simulink model "Boeing787_NewMission_ElectricalThermal"  (R2016a)
(part 7 of 17)

      | value = get_param(blk,'vel') ;
      | cellarr = get_param(blk,'MaskVisibilities') ;
      | ind = [1 4 9 12 15 18 21 24 27 30 33 38 43] ;
      | if strcmp(value,'on')
      |     cellarr(ind) = {'off'} ; cellarr(33:37) = {'on'} ;
      |     value1 = get_param(blk,'fromlen') ;
      |     value2 = get_param(blk,'fromtime') ;
      |     value3 = get_param(blk,'tolen') ;
      |     value4 = get_param(blk,'totime') ;
      |     if strcmp(get_param(blk,'vel'),'on')
      |         switch value1
      |             case 'Millimeters'
      |                 name1 = 'mm/' ;
      |                 fcn1  = 'u(1)/1000' ;
      |             case 'Meters'
      |                 name1 = 'm/' ;
      |                 fcn1  = 'u(1)' ;
      |             case 'Kilometers'
      |                 name1 = 'km/' ;
      |                 fcn1  = 'u(1)*1000' ;
      |             case 'Inches'
      |                 name1 = 'in/' ;
      |                 fcn1  = 'u(1)/39.37008' ;
      |             case 'Feet'
      |                 name1 = 'ft/' ;
      |                 fcn1  = 'u(1)/3.28084';
      |             case 'Yards'
      |                 name1 = 'yd/' ;
      |                 fcn1  = 'u(1)*3/3.28084' ;
      |             case 'Miles'
      |                 name1 = 'mi/' ;
      |                 fcn1  = 'u(1)*1609.344' ;
      |             case 'Nautical Miles'
      |                 name1 = 'nmi/' ;
      |                 fcn1  = 'u(1)*1852' ;
      |         end
      |         switch value2
      |             case 'Millisecond'
      |                 name2 = 'ms' ;
      |                 fcn2  = '*1000'  ;
      |             case 'Second'
      |                 name2 = 's' ;
      |                 fcn2  = '' ;
      |             case 'Minute'
      |                 name2 = 'min' ;
      |                 fcn2  = '/60' ;
      |             case 'Hour'
      |                 name2 = 'hr' ;
      |                 fcn2  = '/3600' ;
      |         end
      |         switch value3
      |             case 'Millimeters'
      |                 name3 = 'mm/' ;
      |                 fcn3  = '*1000' ;
      |             case 'Meters'
      |                 name3 = 'm/' ;
      |                 fcn3  = '' ;
      |             case 'Kilometers'
      |                 name3 = 'km/' ;
      |                 fcn3  = '/1000' ;
      |             case 'Inches'
      |                 name3 = 'in/' ;
      |                 fcn3  = '*39.37008' ;
      |             case 'Feet'
      |                 name3 = 'ft/' ;
      |                 fcn3  = '*3.28084';
      |             case 'Yards'
      |                 name3 = 'yd/' ;
      |                 fcn3  = '/3*3.28084' ;
      |             case 'Miles'
      |                 name3 = 'mi/' ;
      |                 fcn3  = '/1609.344' ;
      |             case 'Nautical Miles'
      |                 name3 = 'nmi/' ;
      |                 fcn3  = '/1852' ;
      |         end
      |         switch value4
      |             case 'Millisecond'
      |                 name4 = 'ms' ;
      |                 fcn4  = '/1000'  ;
      |             case 'Second'
      |                 name4 = 's' ;
      |                 fcn4  = '' ;
      |             case 'Minute'
      |                 name4 = 'min' ;
      |                 fcn4  = '*60' ;
      |             case 'Hour'
      |                 name4 = 'hr' ;
      |                 fcn4  = '*3600' ;
      |         end
      |         expr = [fcn1 fcn2 fcn3 fcn4] ;
      |         %set_param(blk,'func',func) ;
      |         set_param([blk '/conv_fcn'],'expr',expr) ;
      |         str1 = ['% this block of text is updated via dialog callbacks'];
      |         str2 = [char(39) 'horizontalAlignment' char(39) ',' char(39) 'center' char(39) ',' char(39) 'texmode' char(39) ',' char(39) 'on' char(39)] ;
      |         name = [char(39) name1 name2 ' to ' name3 name4 char(39)] ;
      |         str = sprintf('%s\ntext(.5,.5,%s,%s)',str1,name,str2) ;
      |         set_param(blk,'MaskDisplay',str) ;
      |     end
      |     clear value1 value2 value3 value4 expr name1 name2 name3 name4 name fcn1 fcn2 fcn3 fcn4 str1 str2 str
      | 
      | else
      |     cellarr(34:37) = {'off'} ; val = get_param(blk,'MaskValues') ;
      |     for i=1:length(ind)
      |         a = findstr(val{ind(i)},'on') ;
      |         b(i) = isempty(a) ;
      |     end
      |     if isempty(find(b==0)) ;
      |         cellarr(ind) = {'on'} ;
      |     end
      | end
      | set_param(blk,'MaskVisibilities',cellarr) ;
      | clear blk value cellarr ind a b val i
      mask TypeOptions fromlen: Millimeters | Meters | Kilometers | Inches | Feet | Yards | Miles | Nautical Miles
      mask Callback fromlen:
      | blk = gcb ;
      | value1 = get_param(blk,'fromlen') ;
      | value2 = get_param(blk,'fromtime') ;
      | value3 = get_param(blk,'tolen') ;
      | value4 = get_param(blk,'totime') ;
      | if strcmp(get_param(blk,'vel'),'on')
      |     switch value1
      |         case 'Millimeters'
      |             name1 = 'mm/' ;
      |             fcn1  = 'u(1)/1000' ;
      |         case 'Meters'
      |             name1 = 'm/' ;
      |             fcn1  = 'u(1)' ;
      |         case 'Kilometers'
      |             name1 = 'km/' ;
      |             fcn1  = 'u(1)*1000' ;
      |         case 'Inches'
      |             name1 = 'in/' ;
      |             fcn1  = 'u(1)/39.37008' ;
      |         case 'Feet'
      |             name1 = 'ft/' ;
      |             fcn1  = 'u(1)/3.28084';
      |         case 'Yards'
      |             name1 = 'yd/' ;
      |             fcn1  = 'u(1)*3/3.28084' ;
      |         case 'Miles'
      |             name1 = 'mi/' ;
      |             fcn1  = 'u(1)*1609.344' ;
      |         case 'Nautical Miles'
      |             name1 = 'nmi/' ;
      |             fcn1  = 'u(1)*1852' ;
      |     end
      |     switch value2
      |         case 'Millisecond'
      |             name2 = 'ms' ;
      |             fcn2  = '*1000'  ;
      |         case 'Second'
      |             name2 = 's' ;
      |             fcn2  = '' ;
      |         case 'Minute'
      |             name2 = 'min' ;
      |             fcn2  = '/60' ;
      |         case 'Hour'
      |             name2 = 'hr' ;
      |             fcn2  = '/3600' ;
      |     end
      |     switch value3
      |         case 'Millimeters'
      |             name3 = 'mm/' ;
      |             fcn3  = '*1000' ;
      |         case 'Meters'
      |             name3 = 'm/' ;
      |             fcn3  = '' ;
      |         case 'Kilometers'
      |             name3 = 'km/' ;
      |             fcn3  = '/1000' ;
      |         case 'Inches'
      |             name3 = 'in/' ;
      |             fcn3  = '*39.37008' ;
      |         case 'Feet'
      |             name3 = 'ft/' ;
      |             fcn3  = '*3.28084';
      |         case 'Yards'
      |             name3 = 'yd/' ;
      |             fcn3  = '/3*3.28084' ;
      |         case 'Miles'
      |             name3 = 'mi/' ;
      |             fcn3  = '/1609.344' ;
      |         case 'Nautical Miles'
      |             name3 = 'nmi/' ;
      |             fcn3  = '/1852' ;
      |     end
      |     switch value4
      |         case 'Millisecond'
      |             name4 = 'ms' ;
      |             fcn4  = '/1000'  ;
      |         case 'Second'
      |             name4 = 's' ;
      |             fcn4  = '' ;
      |         case 'Minute'
      |             name4 = 'min' ;
      |             fcn4  = '*60' ;
      |         case 'Hour'
      |             name4 = 'hr' ;
      |             fcn4  = '*3600' ;
      |     end
      |     expr = [fcn1 fcn2 fcn3 fcn4] ;
      |     %set_param(blk,'func',func) ;
      |     set_param([blk '/conv_fcn'],'expr',expr) ;
      |     str1 = ['% this block of text is updated via dialog callbacks'];
      |     str2 = [char(39) 'horizontalAlignment' char(39) ',' char(39) 'center' char(39) ',' char(39) 'texmode' char(39) ',' char(39) 'on' char(39)] ;
      |     name = [char(39) name1 name2 ' to ' name3 name4 char(39)] ;
      |     str = sprintf('%s\ntext(.5,.5,%s,%s)',str1,name,str2) ;
      |     set_param(blk,'MaskDisplay',str) ;
      | end
      | clear blk value1 value2 value3 value4 expr name1 name2 name3 name4 name fcn1 fcn2 fcn3 fcn4 str1 str2 str
      mask TypeOptions fromtime: Millisecond | Second | Minute | Hour
      mask Callback fromtime:
      | blk = gcb ;
      | value1 = get_param(blk,'fromlen') ;
      | value2 = get_param(blk,'fromtime') ;
      | value3 = get_param(blk,'tolen') ;
      | value4 = get_param(blk,'totime') ;
      | if strcmp(get_param(blk,'vel'),'on')
      |     switch value1
      |         case 'Millimeters'
      |             name1 = 'mm/' ;
      |             fcn1  = 'u(1)/1000' ;
      |         case 'Meters'
      |             name1 = 'm/' ;
      |             fcn1  = 'u(1)' ;
      |         case 'Kilometers'
      |             name1 = 'km/' ;
      |             fcn1  = 'u(1)*1000' ;
      |         case 'Inches'
      |             name1 = 'in/' ;
      |             fcn1  = 'u(1)/39.37008' ;
      |         case 'Feet'
      |             name1 = 'ft/' ;
      |             fcn1  = 'u(1)/3.28084';
      |         case 'Yards'
      |             name1 = 'yd/' ;
      |             fcn1  = 'u(1)*3/3.28084' ;
      |         case 'Miles'
      |             name1 = 'mi/' ;
      |             fcn1  = 'u(1)*1609.344' ;
      |         case 'Nautical Miles'
      |             name1 = 'nmi/' ;
      |             fcn1  = 'u(1)*1852' ;
      |     end
      |     switch value2
      |         case 'Millisecond'
      |             name2 = 'ms' ;
      |             fcn2  = '*1000'  ;
      |         case 'Second'
      |             name2 = 's' ;
      |             fcn2  = '' ;
      |         case 'Minute'
      |             name2 = 'min' ;
      |             fcn2  = '/60' ;
      |         case 'Hour'
      |             name2 = 'hr' ;
      |             fcn2  = '/3600' ;
      |     end
      |     switch value3
      |         case 'Millimeters'
      |             name3 = 'mm/' ;
      |             fcn3  = '*1000' ;
      |         case 'Meters'
      |             name3 = 'm/' ;
      |             fcn3  = '' ;
      |         case 'Kilometers'
      |             name3 = 'km/' ;
      |             fcn3  = '/1000' ;
      |         case 'Inches'
      |             name3 = 'in/' ;
      |             fcn3  = '*39.37008' ;
      |         case 'Feet'
      |             name3 = 'ft/' ;
      |             fcn3  = '*3.28084';
      |         case 'Yards'
      |             name3 = 'yd/' ;
      |             fcn3  = '/3*3.28084' ;
      |         case 'Miles'
      |             name3 = 'mi/' ;
      |             fcn3  = '/1609.344' ;
      |         case 'Nautical Miles'
      |             name3 = 'nmi/' ;
      |             fcn3  = '/1852' ;
      |     end
      |     switch value4
      |         case 'Millisecond'
      |             name4 = 'ms' ;
      |             fcn4  = '/1000'  ;
      |         case 'Second'
      |             name4 = 's' ;
      |             fcn4  = '' ;
      |         case 'Minute'
      |             name4 = 'min' ;
      |             fcn4  = '*60' ;
      |         case 'Hour'
      |             name4 = 'hr' ;
      |             fcn4  = '*3600' ;
      |     end
      |     expr = [fcn1 fcn2 fcn3 fcn4] ;
      |     %set_param(blk,'func',func) ;
      |     set_param([blk '/conv_fcn'],'expr',expr) ;
      |     str1 = ['% this block of text is updated via dialog callbacks'];
      |     str2 = [char(39) 'horizontalAlignment' char(39) ',' char(39) 'center' char(39) ',' char(39) 'texmode' char(39) ',' char(39) 'on' char(39)] ;
      |     name = [char(39) name1 name2 ' to ' name3 name4 char(39)] ;
      |     str = sprintf('%s\ntext(.5,.5,%s,%s)',str1,name,str2) ;
      |     set_param(blk,'MaskDisplay',str) ;
      | end
      | clear blk value1 value2 value3 value4 expr name1 name2 name3 name4 name fcn1 fcn2 fcn3 fcn4 str1 str2 str
      mask TypeOptions tolen: Millimeters | Meters | Kilometers | Inches | Feet | Yards | Miles | Nautical Miles
      mask Callback tolen:
      | blk = gcb ;
      | value1 = get_param(blk,'fromlen') ;
      | value2 = get_param(blk,'fromtime') ;
      | value3 = get_param(blk,'tolen') ;
      | value4 = get_param(blk,'totime') ;
      | if strcmp(get_param(blk,'vel'),'on')
      |     switch value1
      |         case 'Millimeters'
      |             name1 = 'mm/' ;
      |             fcn1  = 'u(1)/1000' ;
      |         case 'Meters'
      |             name1 = 'm/' ;
      |             fcn1  = 'u(1)' ;
      |         case 'Kilometers'
      |             name1 = 'km/' ;
      |             fcn1  = 'u(1)*1000' ;
      |         case 'Inches'
      |             name1 = 'in/' ;
      |             fcn1  = 'u(1)/39.37008' ;
      |         case 'Feet'
      |             name1 = 'ft/' ;
      |             fcn1  = 'u(1)/3.28084';
      |         case 'Yards'
      |             name1 = 'yd/' ;
      |             fcn1  = 'u(1)*3/3.28084' ;
      |         case 'Miles'
      |             name1 = 'mi/' ;
      |             fcn1  = 'u(1)*1609.344' ;
      |         case 'Nautical Miles'
      |             name1 = 'nmi/' ;
      |             fcn1  = 'u(1)*1852' ;
      |     end
      |     switch value2
      |         case 'Millisecond'
      |             name2 = 'ms' ;
      |             fcn2  = '*1000'  ;
      |         case 'Second'
      |             name2 = 's' ;
      |             fcn2  = '' ;
      |         case 'Minute'
      |             name2 = 'min' ;
      |             fcn2  = '/60' ;
      |         case 'Hour'
      |             name2 = 'hr' ;
      |             fcn2  = '/3600' ;
      |     end
      |     switch value3
      |         case 'Millimeters'
      |             name3 = 'mm/' ;
      |             fcn3  = '*1000' ;
      |         case 'Meters'
      |             name3 = 'm/' ;
      |             fcn3  = '' ;
      |         case 'Kilometers'
      |             name3 = 'km/' ;
      |             fcn3  = '/1000' ;
      |         case 'Inches'
      |             name3 = 'in/' ;
      |             fcn3  = '*39.37008' ;
      |         case 'Feet'
      |             name3 = 'ft/' ;
      |             fcn3  = '*3.28084';
      |         case 'Yards'
      |             name3 = 'yd/' ;
      |             fcn3  = '/3*3.28084' ;
      |         case 'Miles'
      |             name3 = 'mi/' ;
      |             fcn3  = '/1609.344' ;
      |         case 'Nautical Miles'
      |             name3 = 'nmi/' ;
      |             fcn3  = '/1852' ;
      |     end
      |     switch value4
      |         case 'Millisecond'
      |             name4 = 'ms' ;
      |             fcn4  = '/1000'  ;
      |         case 'Second'
      |             name4 = 's' ;
      |             fcn4  = '' ;
      |         case 'Minute'
      |             name4 = 'min' ;
      |             fcn4  = '*60' ;
      |         case 'Hour'
      |             name4 = 'hr' ;
      |             fcn4  = '*3600' ;
      |     end
      |     expr = [fcn1 fcn2 fcn3 fcn4] ;
      |     %set_param(blk,'func',func) ;
      |     set_param([blk '/conv_fcn'],'expr',expr) ;
      |     str1 = ['% this block of text is updated via dialog callbacks'];
      |     str2 = [char(39) 'horizontalAlignment' char(39) ',' char(39) 'center' char(39) ',' char(39) 'texmode' char(39) ',' char(39) 'on' char(39)] ;
      |     name = [char(39) name1 name2 ' to ' name3 name4 char(39)] ;
      |     str = sprintf('%s\ntext(.5,.5,%s,%s)',str1,name,str2) ;
      |     set_param(blk,'MaskDisplay',str) ;
      | end
      | clear blk value1 value2 value3 value4 expr name1 name2 name3 name4 name fcn1 fcn2 fcn3 fcn4 str1 str2 str
      mask TypeOptions totime: Millisecond | Second | Minute | Hour
      mask Callback totime:
      | blk = gcb ;
      | value1 = get_param(blk,'fromlen') ;
      | value2 = get_param(blk,'fromtime') ;
      | value3 = get_param(blk,'tolen') ;
      | value4 = get_param(blk,'totime') ;
      | if strcmp(get_param(blk,'vel'),'on')
      |     switch value1
      |         case 'Millimeters'
      |             name1 = 'mm/' ;
      |             fcn1  = 'u(1)/1000' ;
      |         case 'Meters'
      |             name1 = 'm/' ;
      |             fcn1  = 'u(1)' ;
      |         case 'Kilometers'
      |             name1 = 'km/' ;
      |             fcn1  = 'u(1)*1000' ;
      |         case 'Inches'
      |             name1 = 'in/' ;
      |             fcn1  = 'u(1)/39.37008' ;
      |         case 'Feet'
      |             name1 = 'ft/' ;
      |             fcn1  = 'u(1)/3.28084';
      |         case 'Yards'
      |             name1 = 'yd/' ;
      |             fcn1  = 'u(1)*3/3.28084' ;
      |         case 'Miles'
      |             name1 = 'mi/' ;
      |             fcn1  = 'u(1)*1609.344' ;
      |         case 'Nautical Miles'
      |             name1 = 'nmi/' ;
      |             fcn1  = 'u(1)*1852' ;
      |     end
      |     switch value2
      |         case 'Millisecond'
      |             name2 = 'ms' ;
      |             fcn2  = '*1000'  ;
      |         case 'Second'
      |             name2 = 's' ;
      |             fcn2  = '' ;
      |         case 'Minute'
      |             name2 = 'min' ;
      |             fcn2  = '/60' ;
      |         case 'Hour'
      |             name2 = 'hr' ;
      |             fcn2  = '/3600' ;
      |     end
      |     switch value3
      |         case 'Millimeters'
      |             name3 = 'mm/' ;
      |             fcn3  = '*1000' ;
      |         case 'Meters'
      |             name3 = 'm/' ;
      |             fcn3  = '' ;
      |         case 'Kilometers'
      |             name3 = 'km/' ;
      |             fcn3  = '/1000' ;
      |         case 'Inches'
      |             name3 = 'in/' ;
      |             fcn3  = '*39.37008' ;
      |         case 'Feet'
      |             name3 = 'ft/' ;
      |             fcn3  = '*3.28084';
      |         case 'Yards'
      |             name3 = 'yd/' ;
      |             fcn3  = '/3*3.28084' ;
      |         case 'Miles'
      |             name3 = 'mi/' ;
      |             fcn3  = '/1609.344' ;
      |         case 'Nautical Miles'
      |             name3 = 'nmi/' ;
      |             fcn3  = '/1852' ;
      |     end
      |     switch value4
      |         case 'Millisecond'
      |             name4 = 'ms' ;
      |             fcn4  = '/1000'  ;
      |         case 'Second'
      |             name4 = 's' ;
      |             fcn4  = '' ;
      |         case 'Minute'
      |             name4 = 'min' ;
      |             fcn4  = '*60' ;
      |         case 'Hour'
      |             name4 = 'hr' ;
      |             fcn4  = '*3600' ;
      |     end
      |     expr = [fcn1 fcn2 fcn3 fcn4] ;
      |     %set_param(blk,'func',func) ;
      |     set_param([blk '/conv_fcn'],'expr',expr) ;
      |     str1 = ['% this block of text is updated via dialog callbacks'];
      |     str2 = [char(39) 'horizontalAlignment' char(39) ',' char(39) 'center' char(39) ',' char(39) 'texmode' char(39) ',' char(39) 'on' char(39)] ;
      |     name = [char(39) name1 name2 ' to ' name3 name4 char(39)] ;
      |     str = sprintf('%s\ntext(.5,.5,%s,%s)',str1,name,str2) ;
      |     set_param(blk,'MaskDisplay',str) ;
      | end
      | clear blk value1 value2 value3 value4 expr name1 name2 name3 name4 name fcn1 fcn2 fcn3 fcn4 str1 str2 str
      mask Callback flow_rate:
      | blk = gcb ;
      | value = get_param(blk,'flow_rate') ;
      | cellarr = get_param(blk,'MaskVisibilities') ;
      | ind = [1 4 9 12 15 18 21 24 27 30 33 38 43] ;
      | if strcmp(value,'on')
      |     cellarr(ind) = {'off'} ; cellarr(38:42) = {'on'} ;
      |     value1 = get_param(blk,'fromflowvol') ;
      |     value2 = get_param(blk,'fromflvoltime') ;
      |     value3 = get_param(blk,'toflowvol') ;
      |     value4 = get_param(blk,'toflvoltime') ;
      |     if strcmp(get_param(blk,'flow_rate'),'on')
      |         switch value1
      |             case 'Milliliters'
      |                 name1 = 'mL/' ;
      |                 fcn1  = 'u(1)*(1e-6)' ;
      |             case 'Liters'
      |                 name1 = 'L/' ;
      |                 fcn1  = 'u(1)*.001' ;
      |             case 'Cubic Centimeters'
      |                 name1 = 'cm^3/' ;
      |                 fcn1  = 'u(1)*(1e-6)' ;
      |             case 'Cubic Meters'
      |                 name1 = 'm^3/' ;
      |                 fcn1  = 'u(1)' ;
      |             case 'Ounces'
      |                 name1 = 'oz/' ;
      |                 fcn1  = 'u(1)*(2.957353e-5)';
      |             case 'Gallons'
      |                 name1 = 'gal/' ;
      |                 fcn1  = 'u(1)*.00378541' ;
      |             case 'Cubic Inches'
      |                 name1 = 'in^3/' ;
      |                 fcn1  = 'u(1)*(1.6387e-5)' ;
      |             case 'Cubic Feet'
      |                 name1 = 'ft^3/' ;
      |                 fcn1  = 'u(1)*.0283168' ;
      |         end
      |         switch value2
      |             case 'Millisecond'
      |                 name2 = 'ms' ;
      |                 fcn2  = '*1000'  ;
      |             case 'Second'
      |                 name2 = 's' ;
      |                 fcn2  = '' ;
      |             case 'Minute'
      |                 name2 = 'min' ;
      |                 fcn2  = '/60' ;
      |             case 'Hour'
      |                 name2 = 'hr' ;
      |                 fcn2  = '/3600' ;
      |         end
      |         switch value3
      |             case 'Milliliters'
      |                 name3 = 'mL/' ;
      |                 fcn3  = '/(1e-6)' ;
      |             case 'Liters'
      |                 name3 = 'L/' ;
      |                 fcn3  = '/.001' ;
      |             case 'Cubic Centimeters'
      |                 name3 = 'cm^3/' ;
      |                 fcn3  = '/(1e-6)' ;
      |             case 'Cubic Meters'
      |                 name3 = 'm^3/' ;
      |                 fcn3  = '' ;
      |             case 'Ounces'
      |                 name3 = 'oz/' ;
      |                 fcn3  = '/(2.957353e-5)';
      |             case 'Gallons'
      |                 name3 = 'gal/' ;
      |                 fcn3  = '/.00378541' ;
      |             case 'Cubic Inches'
      |                 name3 = 'in^3/' ;
      |                 fcn3  = '/(1.6387e-5)' ;
      |             case 'Cubic Feet'
      |                 name3 = 'ft^3/' ;
      |                 fcn3  = '/.0283168' ;
      |         end
      |         switch value4
      |             case 'Millisecond'
      |                 name4 = 'ms' ;
      |                 fcn4  = '/1000'  ;
      |             case 'Second'
      |                 name4 = 's' ;
      |                 fcn4  = '' ;
      |             case 'Minute'
      |                 name4 = 'min' ;
      |                 fcn4  = '*60' ;
      |             case 'Hour'
      |                 name4 = 'hr' ;
      |                 fcn4  = '*3600' ;
      |         end
      |         expr = [fcn1 fcn2 fcn3 fcn4] ;
      |         %set_param(blk,'func',func) ;
      |         set_param([blk '/conv_fcn'],'expr',expr) ;
      |         str1 = ['% this block of text is updated via dialog callbacks'];
      |         str2 = [char(39) 'horizontalAlignment' char(39) ',' char(39) 'center' char(39) ',' char(39) 'texmode' char(39) ',' char(39) 'on' char(39)] ;
      |         name = [char(39) name1 name2 ' to ' name3 name4 char(39)] ;
      |         str = sprintf('%s\ntext(.5,.5,%s,%s)',str1,name,str2) ;
      |         set_param(blk,'MaskDisplay',str) ;
      |     end
      |     clear value1 value2 value3 value4 expr name1 name2 name3 name4 name fcn1 fcn2 fcn3 fcn4 str1 str2 str
      | else
      |     cellarr(39:42) = {'off'} ; val = get_param(blk,'MaskValues') ;
      |     for i=1:length(ind)
      |         a = findstr(val{ind(i)},'on') ;
      |         b(i) = isempty(a) ;
      |     end
      |     if isempty(find(b==0)) ;
      |         cellarr(ind) = {'on'} ;
      |     end
      | end
      | set_param(blk,'MaskVisibilities',cellarr) ;
      | clear blk value cellarr ind a b val i
      mask TypeOptions fromflowvol: Milliliters | Liters | Cubic Centimeters | Cubic Meters | Ounces | Gallons | Cubic Inches | Cubic Feet
      mask Callback fromflowvol:
      | blk = gcb ;
      | value1 = get_param(blk,'fromflowvol') ;
      | value2 = get_param(blk,'fromflvoltime') ;
      | value3 = get_param(blk,'toflowvol') ;
      | value4 = get_param(blk,'toflvoltime') ;
      | if strcmp(get_param(blk,'flow_rate'),'on')
      |     switch value1
      |         case 'Milliliters'
      |             name1 = 'mL/' ;
      |             fcn1  = 'u(1)*(1e-6)';
      |         case 'Liters'
      |             name1 = 'L/' ;
      |             fcn1  = 'u(1)*.001' ;
      |         case 'Cubic Centimeters'
      |             name1 = 'cm^3/' ;
      |             fcn1  = 'u(1)*(1e-6)' ;
      |         case 'Cubic Meters'
      |             name1 = 'm^3/' ;
      |             fcn1  = 'u(1)' ;
      |         case 'Ounces'
      |             name1 = 'oz/' ;
      |             fcn1  = 'u(1)*(2.957353e-5)';
      |         case 'Gallons'
      |             name1 = 'gal/' ;
      |             fcn1  = 'u(1)*.00378541' ;
      |         case 'Cubic Inches'
      |             name1 = 'in^3/' ;
      |             fcn1  = 'u(1)*(1.6387e-5)' ;
      |         case 'Cubic Feet'
      |             name1 = 'ft^3/' ;
      |             fcn1  = 'u(1)*.0283168' ;
      |     end
      |     switch value2
      |         case 'Millisecond'
      |             name2 = 'ms' ;
      |             fcn2  = '*1000'  ;
      |         case 'Second'
      |             name2 = 's' ;
      |             fcn2  = '' ;
      |         case 'Minute'
      |             name2 = 'min' ;
      |             fcn2  = '/60' ;
      |         case 'Hour'
      |             name2 = 'hr' ;
      |             fcn2  = '/3600' ;
      |     end
      |     switch value3
      |         case 'Milliliters'
      |             name3 = 'mL/' ;
      |             fcn3  = '/(1e-6)' ;
      |         case 'Liters'
      |             name3 = 'L/' ;
      |             fcn3  = '/.001' ;
      |         case 'Cubic Centimeters'
      |             name3 = 'cm^3/' ;
      |             fcn3  = '/(1e-6)' ;
      |         case 'Cubic Meters'
      |             name3 = 'm^3/' ;
      |             fcn3  = '' ;
      |         case 'Ounces'
      |             name3 = 'oz/' ;
      |             fcn3  = '/(2.957353e-5)';
      |         case 'Gallons'
      |             name3 = 'gal/' ;
      |             fcn3  = '/.00378541' ;
      |         case 'Cubic Inches'
      |             name3 = 'in^3/' ;
      |             fcn3  = '/(1.6387e-5)' ;
      |         case 'Cubic Feet'
      |             name3 = 'ft^3/' ;
      |             fcn3  = '/.0283168' ;
      |     end
      |     switch value4
      |         case 'Millisecond'
      |             name4 = 'ms' ;
      |             fcn4  = '/1000'  ;
      |         case 'Second'
      |             name4 = 's' ;
      |             fcn4  = '' ;
      |         case 'Minute'
      |             name4 = 'min' ;
      |             fcn4  = '*60' ;
      |         case 'Hour'
      |             name4 = 'hr' ;
      |             fcn4  = '*3600' ;
      |     end
      |     expr = [fcn1 fcn2 fcn3 fcn4] ;
      |     %set_param(blk,'func',func) ;
      |     set_param([blk '/conv_fcn'],'expr',expr) ;
      |     str1 = ['% this block of text is updated via dialog callbacks'];
      |     str2 = [char(39) 'horizontalAlignment' char(39) ',' char(39) 'center' char(39) ',' char(39) 'texmode' char(39) ',' char(39) 'on' char(39)] ;
      |     name = [char(39) name1 name2 ' to ' name3 name4 char(39)] ;
      |     str = sprintf('%s\ntext(.5,.5,%s,%s)',str1,name,str2) ;
      |     set_param(blk,'MaskDisplay',str) ;
      | end
      | clear blk value1 value2 value3 value4 expr name1 name2 name3 name4 name fcn1 fcn2 fcn3 fcn4 str1 str2 str
      mask TypeOptions fromflvoltime: Millisecond | Second | Minute | Hour
      mask Callback fromflvoltime:
      | blk = gcb ;
      | value1 = get_param(blk,'fromflowvol') ;
      | value2 = get_param(blk,'fromflvoltime') ;
      | value3 = get_param(blk,'toflowvol') ;
      | value4 = get_param(blk,'toflvoltime') ;
      | if strcmp(get_param(blk,'flow_rate'),'on')
      |     switch value1
      |         case 'Milliliters'
      |             name1 = 'mL/' ;
      |             fcn1  = 'u(1)*(1e-6)' ;
      |         case 'Liters'
      |             name1 = 'L/' ;
      |             fcn1  = 'u(1)*.001' ;
      |         case 'Cubic Centimeters'
      |             name1 = 'cm^3/' ;
      |             fcn1  = 'u(1)*(1e-6)' ;
      |         case 'Cubic Meters'
      |             name1 = 'm^3/' ;
      |             fcn1  = 'u(1)' ;
      |         case 'Ounces'
      |             name1 = 'oz/' ;
      |             fcn1  = 'u(1)*(2.957353e-5)';
      |         case 'Gallons'
      |             name1 = 'gal/' ;
      |             fcn1  = 'u(1)*.00378541' ;
      |         case 'Cubic Inches'
      |             name1 = 'in^3/' ;
      |             fcn1  = 'u(1)*(1.6387e-5)' ;
      |         case 'Cubic Feet'
      |             name1 = 'ft^3/' ;
      |             fcn1  = 'u(1)*.0283168' ;
      |     end
      |     switch value2
      |         case 'Millisecond'
      |             name2 = 'ms' ;
      |             fcn2  = '*1000'  ;
      |         case 'Second'
      |             name2 = 's' ;
      |             fcn2  = '' ;
      |         case 'Minute'
      |             name2 = 'min' ;
      |             fcn2  = '/60' ;
      |         case 'Hour'
      |             name2 = 'hr' ;
      |             fcn2  = '/3600' ;
      |     end
      |     switch value3
      |         case 'Milliliters'
      |             name3 = 'mL/' ;
      |             fcn3  = '/(1e-6)' ;
      |         case 'Liters'
      |             name3 = 'L/' ;
      |             fcn3  = '/.001' ;
      |         case 'Cubic Centimeters'
      |             name3 = 'cm^3/' ;
      |             fcn3  = '/(1e-6)' ;
      |         case 'Cubic Meters'
      |             name3 = 'm^3/' ;
      |             fcn3  = '' ;
      |         case 'Ounces'
      |             name3 = 'oz/' ;
      |             fcn3  = '/(2.957353e-5)';
      |         case 'Gallons'
      |             name3 = 'gal/' ;
      |             fcn3  = '/.00378541' ;
      |         case 'Cubic Inches'
      |             name3 = 'in^3/' ;
      |             fcn3  = '/(1.6387e-5)' ;
      |         case 'Cubic Feet'
      |             name3 = 'ft^3/' ;
      |             fcn3  = '/.0283168' ;
      |     end
      |     switch value4
      |         case 'Millisecond'
      |             name4 = 'ms' ;
      |             fcn4  = '/1000'  ;
      |         case 'Second'
      |             name4 = 's' ;
      |             fcn4  = '' ;
      |         case 'Minute'
      |             name4 = 'min' ;
      |             fcn4  = '*60' ;
      |         case 'Hour'
      |             name4 = 'hr' ;
      |             fcn4  = '*3600' ;
      |     end
      |     expr = [fcn1 fcn2 fcn3 fcn4] ;
      |     %set_param(blk,'func',func) ;
      |     set_param([blk '/conv_fcn'],'expr',expr) ;
      |     str1 = ['% this block of text is updated via dialog callbacks'];
      |     str2 = [char(39) 'horizontalAlignment' char(39) ',' char(39) 'center' char(39) ',' char(39) 'texmode' char(39) ',' char(39) 'on' char(39)] ;
      |     name = [char(39) name1 name2 ' to ' name3 name4 char(39)] ;
      |     str = sprintf('%s\ntext(.5,.5,%s,%s)',str1,name,str2) ;
      |     set_param(blk,'MaskDisplay',str) ;
      | end
      | clear blk value1 value2 value3 value4 expr name1 name2 name3 name4 name fcn1 fcn2 fcn3 fcn4 str1 str2 str
      mask TypeOptions toflowvol: Milliliters | Liters | Cubic Centimeters | Cubic Meters | Ounces | Gallons | Cubic Inches | Cubic Feet
      mask Callback toflowvol:
      | blk = gcb ;
      | value1 = get_param(blk,'fromflowvol') ;
      | value2 = get_param(blk,'fromflvoltime') ;
      | value3 = get_param(blk,'toflowvol') ;
      | value4 = get_param(blk,'toflvoltime') ;
      | if strcmp(get_param(blk,'flow_rate'),'on')
      |     switch value1
      |         case 'Milliliters'
      |             name1 = 'mL/' ;
      |             fcn1  = 'u(1)*(1e-6)' ;
      |         case 'Liters'
      |             name1 = 'L/' ;
      |             fcn1  = 'u(1)*.001' ;
      |         case 'Cubic Centimeters'
      |             name1 = 'cm^3/' ;
      |             fcn1  = 'u(1)*(1e-6)' ;
      |         case 'Cubic Meters'
      |             name1 = 'm^3/' ;
      |             fcn1  = 'u(1)' ;
      |         case 'Ounces'
      |             name1 = 'oz/' ;
      |             fcn1  = 'u(1)*(2.957353e-5)';
      |         case 'Gallons'
      |             name1 = 'gal/' ;
      |             fcn1  = 'u(1)*.00378541' ;
      |         case 'Cubic Inches'
      |             name1 = 'in^3/' ;
      |             fcn1  = 'u(1)*(1.6387e-5)' ;
      |         case 'Cubic Feet'
      |             name1 = 'ft^3/' ;
      |             fcn1  = 'u(1)*.0283168' ;
      |     end
      |     switch value2
      |         case 'Millisecond'
      |             name2 = 'ms' ;
      |             fcn2  = '*1000'  ;
      |         case 'Second'
      |             name2 = 's' ;
      |             fcn2  = '' ;
      |         case 'Minute'
      |             name2 = 'min' ;
      |             fcn2  = '/60' ;
      |         case 'Hour'
      |             name2 = 'hr' ;
      |             fcn2  = '/3600' ;
      |     end
      |     switch value3
      |         case 'Milliliters'
      |             name3 = 'mL/' ;
      |             fcn3  = '/(1e-6)' ;
      |         case 'Liters'
      |             name3 = 'L/' ;
      |             fcn3  = '/.001' ;
      |         case 'Cubic Centimeters'
      |             name3 = 'cm^3/' ;
      |             fcn3  = '/(1e-6)' ;
      |         case 'Cubic Meters'
      |             name3 = 'm^3/' ;
      |             fcn3  = '' ;
      |         case 'Ounces'
      |             name3 = 'oz/' ;
      |             fcn3  = '/(2.957353e-5)';
      |         case 'Gallons'
      |             name3 = 'gal/' ;
      |             fcn3  = '/.00378541' ;
      |         case 'Cubic Inches'
      |             name3 = 'in^3/' ;
      |             fcn3  = '/(1.6387e-5)' ;
      |         case 'Cubic Feet'
      |             name3 = 'ft^3/' ;
      |             fcn3  = '/.0283168' ;
      |     end
      |     switch value4
      |         case 'Millisecond'
      |             name4 = 'ms' ;
      |             fcn4  = '/1000'  ;
      |         case 'Second'
      |             name4 = 's' ;
      |             fcn4  = '' ;
      |         case 'Minute'
      |             name4 = 'min' ;
      |             fcn4  = '*60' ;
      |         case 'Hour'
      |             name4 = 'hr' ;
      |             fcn4  = '*3600' ;
      |     end
      |     expr = [fcn1 fcn2 fcn3 fcn4] ;
      |     %set_param(blk,'func',func) ;
      |     set_param([blk '/conv_fcn'],'expr',expr) ;
      |     str1 = ['% this block of text is updated via dialog callbacks'];
      |     str2 = [char(39) 'horizontalAlignment' char(39) ',' char(39) 'center' char(39) ',' char(39) 'texmode' char(39) ',' char(39) 'on' char(39)] ;
      |     name = [char(39) name1 name2 ' to ' name3 name4 char(39)] ;
      |     str = sprintf('%s\ntext(.5,.5,%s,%s)',str1,name,str2) ;
      |     set_param(blk,'MaskDisplay',str) ;
      | end
      | clear blk value1 value2 value3 value4 expr name1 name2 name3 name4 name fcn1 fcn2 fcn3 fcn4 str1 str2 str
      mask TypeOptions toflvoltime: Millisecond | Second | Minute | Hour
      mask Callback toflvoltime:
      | blk = gcb ;
      | value1 = get_param(blk,'fromflowvol') ;
      | value2 = get_param(blk,'fromflvoltime') ;
      | value3 = get_param(blk,'toflowvol') ;
      | value4 = get_param(blk,'toflvoltime') ;
      | if strcmp(get_param(blk,'flow_rate'),'on')
      |     switch value1
      |         case 'Milliliters'
      |             name1 = 'mL/' ;
      |             fcn1  = 'u(1)*(1e-6)' ;
      |         case 'Liters'
      |             name1 = 'L/' ;
      |             fcn1  = 'u(1)*.001' ;
      |         case 'Cubic Centimeters'
      |             name1 = 'cm^3/' ;
      |             fcn1  = 'u(1)*(1e-6)' ;
      |         case 'Cubic Meters'
      |             name1 = 'm^3/' ;
      |             fcn1  = 'u(1)' ;
      |         case 'Ounces'
      |             name1 = 'oz/' ;
      |             fcn1  = 'u(1)*(2.957353e-5)';
      |         case 'Gallons'
      |             name1 = 'gal/' ;
      |             fcn1  = 'u(1)*.00378541' ;
      |         case 'Cubic Inches'
      |             name1 = 'in^3/' ;
      |             fcn1  = 'u(1)*(1.6387e-5)' ;
      |         case 'Cubic Feet'
      |             name1 = 'ft^3/' ;
      |             fcn1  = 'u(1)*.0283168' ;
      |     end
      |     switch value2
      |         case 'Millisecond'
      |             name2 = 'ms' ;
      |             fcn2  = '*1000'  ;
      |         case 'Second'
      |             name2 = 's' ;
      |             fcn2  = '' ;
      |         case 'Minute'
      |             name2 = 'min' ;
      |             fcn2  = '/60' ;
      |         case 'Hour'
      |             name2 = 'hr' ;
      |             fcn2  = '/3600' ;
      |     end
      |     switch value3
      |         case 'Milliliters'
      |             name3 = 'mL/' ;
      |             fcn3  = '/(1e-6)' ;
      |         case 'Liters'
      |             name3 = 'L/' ;
      |             fcn3  = '/.001' ;
      |         case 'Cubic Centimeters'
      |             name3 = 'cm^3/' ;
      |             fcn3  = '/(1e-6)' ;
      |         case 'Cubic Meters'
      |             name3 = 'm^3/' ;
      |             fcn3  = '' ;
      |         case 'Ounces'
      |             name3 = 'oz/' ;
      |             fcn3  = '/(2.957353e-5)';
      |         case 'Gallons'
      |             name3 = 'gal/' ;
      |             fcn3  = '/.00378541' ;
      |         case 'Cubic Inches'
      |             name3 = 'in^3/' ;
      |             fcn3  = '/(1.6387e-5)' ;
      |         case 'Cubic Feet'
      |             name3 = 'ft^3/' ;
      |             fcn3  = '/.0283168' ;
      |     end
      |     switch value4
      |         case 'Millisecond'
      |             name4 = 'ms' ;
      |             fcn4  = '/1000'  ;
      |         case 'Second'
      |             name4 = 's' ;
      |             fcn4  = '' ;
      |         case 'Minute'
      |             name4 = 'min' ;
      |             fcn4  = '*60' ;
      |         case 'Hour'
      |             name4 = 'hr' ;
      |             fcn4  = '*3600' ;
      |     end
      |     expr = [fcn1 fcn2 fcn3 fcn4] ;
      |     %set_param(blk,'func',func) ;
      |     set_param([blk '/conv_fcn'],'expr',expr) ;
      |     str1 = ['% this block of text is updated via dialog callbacks'];
      |     str2 = [char(39) 'horizontalAlignment' char(39) ',' char(39) 'center' char(39) ',' char(39) 'texmode' char(39) ',' char(39) 'on' char(39)] ;
      |     name = [char(39) name1 name2 ' to ' name3 name4 char(39)] ;
      |     str = sprintf('%s\ntext(.5,.5,%s,%s)',str1,name,str2) ;
      |     set_param(blk,'MaskDisplay',str) ;
      | end
      | clear blk value1 value2 value3 value4 expr name1 name2 name3 name4 name fcn1 fcn2 fcn3 fcn4 str1 str2 str
      mask Callback mfr:
      | blk = gcb ;
      | value = get_param(blk,'mfr') ;
      | cellarr = get_param(blk,'MaskVisibilities') ;
      | ind = [1 4 9 12 15 18 21 24 27 30 33 38 43] ;
      | if strcmp(value,'on')
      |     cellarr(ind) = {'off'} ; cellarr(43:47) = {'on'} ;
      |     value1 = get_param(blk,'frommfr') ;
      |     value2 = get_param(blk,'frommfrtime') ;
      |     value3 = get_param(blk,'tomfr') ;
      |     value4 = get_param(blk,'tomfrtime') ;
      |     if strcmp(get_param(blk,'mfr'),'on')
      |         switch value1
      |             case 'Grams'
      |                 name1 = 'g/' ;
      |                 fcn1  = 'u(1)*.001' ;
      |             case 'Kilograms'
      |                 name1 = 'kg/' ;
      |                 fcn1  = 'u(1)' ;
      |             case 'Ounces'
      |                 name1 = 'oz/' ;
      |                 fcn1  = 'u(1)*.45359237/16' ;
      |             case 'Pounds-Mass'
      |                 name1 = 'lbm/' ;
      |                 fcn1  = 'u(1)*.45359237' ;
      |             case 'Slugs'
      |                 name1 = 'slg/' ;
      |                 fcn1  = 'u(1)*14.5939';
      |         end
      |         switch value2
      |             case 'Millisecond'
      |                 name2 = 'ms' ;
      |                 fcn2  = '*1000'  ;
      |             case 'Second'
      |                 name2 = 's' ;
      |                 fcn2  = '' ;
      |             case 'Minute'
      |                 name2 = 'min' ;
      |                 fcn2  = '/60' ;
      |             case 'Hour'
      |                 name2 = 'hr' ;
      |                 fcn2  = '/3600' ;
      |         end
      |         switch value3
      |             case 'Grams'
      |                 name3 = 'g/' ;
      |                 fcn3  = '/.001' ;
      |             case 'Kilograms'
      |                 name3 = 'kg/' ;
      |                 fcn3  = '' ;
      |             case 'Ounces'
      |                 name3 = 'oz/' ;
      |                 fcn3  = '/.45359237*16' ;
      |             case 'Pounds-Mass'
      |                 name3 = 'lbm/' ;
      |                 fcn3  = '/.45359237' ;
      |             case 'Slugs'
      |                 name3 = 'slg/' ;
      |                 fcn3  = '/14.5939';
      |         end
      |         switch value4
      |             case 'Millisecond'
      |                 name4 = 'ms' ;
      |                 fcn4  = '/1000'  ;
      |             case 'Second'
      |                 name4 = 's' ;
      |                 fcn4  = '' ;
      |             case 'Minute'
      |                 name4 = 'min' ;
      |                 fcn4  = '*60' ;
      |             case 'Hour'
      |                 name4 = 'hr' ;
      |                 fcn4  = '*3600' ;
      |         end
      |         expr = [fcn1 fcn2 fcn3 fcn4] ;
      |         %set_param(blk,'func',func) ;
      |         set_param([blk '/conv_fcn'],'expr',expr) ;
      |         str1 = ['% this block of text is updated via dialog callbacks'];
      |         str2 = [char(39) 'horizontalAlignment' char(39) ',' char(39) 'center' char(39) ',' char(39) 'texmode' char(39) ',' char(39) 'on' char(39)] ;
      |         name = [char(39) name1 name2 ' to ' name3 name4 char(39)] ;
      |         str = sprintf('%s\ntext(.5,.5,%s,%s)',str1,name,str2) ;
      |         set_param(blk,'MaskDisplay',str) ;
      |     end
      |     clear value1 value2 value3 value4 expr name1 name2 name3 name4 name fcn1 fcn2 fcn3 fcn4 str1 str2 str
      | else
      |     cellarr(44:47) = {'off'} ; val = get_param(blk,'MaskValues') ;
      |     for i=1:length(ind)
      |         a = findstr(val{ind(i)},'on') ;
      |         b(i) = isempty(a) ;
      |     end
      |     if isempty(find(b==0)) ;
      |         cellarr(ind) = {'on'} ;
      |     end
      | end
      | set_param(blk,'MaskVisibilities',cellarr) ;
      | clear blk value cellarr ind a b val i
      mask TypeOptions frommfr: Grams | Kilograms | Ounces | Pounds-Mass | Slugs
      mask Callback frommfr:
      | blk = gcb ;
      | value1 = get_param(blk,'frommfr') ;
      | value2 = get_param(blk,'frommfrtime') ;
      | value3 = get_param(blk,'tomfr') ;
      | value4 = get_param(blk,'tomfrtime') ;
      | if strcmp(get_param(blk,'mfr'),'on')
      |     switch value1
      |         case 'Grams'
      |             name1 = 'g/' ;
      |             fcn1  = 'u(1)*.001' ;
      |         case 'Kilograms'
      |             name1 = 'kg/' ;
      |             fcn1  = 'u(1)' ;
      |         case 'Ounces'
      |             name1 = 'oz/' ;
      |             fcn1  = 'u(1)*.45359237/16' ;
      |         case 'Pounds-Mass'
      |             name1 = 'lbm/' ;
      |             fcn1  = 'u(1)*.45359237' ;
      |         case 'Slugs'
      |             name1 = 'slg/' ;
      |             fcn1  = 'u(1)*14.5939';
      |     end
      |     switch value2
      |         case 'Millisecond'
      |             name2 = 'ms' ;
      |             fcn2  = '*1000'  ;
      |         case 'Second'
      |             name2 = 's' ;
      |             fcn2  = '' ;
      |         case 'Minute'
      |             name2 = 'min' ;
      |             fcn2  = '/60' ;
      |         case 'Hour'
      |             name2 = 'hr' ;
      |             fcn2  = '/3600' ;
      |     end
      |     switch value3
      |         case 'Grams'
      |             name3 = 'g/' ;
      |             fcn3  = '/.001' ;
      |         case 'Kilograms'
      |             name3 = 'kg/' ;
      |             fcn3  = '' ;
      |         case 'Ounces'
      |             name3 = 'oz/' ;
      |             fcn3  = '/.45359237*16' ;
      |         case 'Pounds-Mass'
      |             name3 = 'lbm/' ;
      |             fcn3  = '/.45359237' ;
      |         case 'Slugs'
      |             name3 = 'slg/' ;
      |             fcn3  = '/14.5939';
      |     end
      |     switch value4
      |         case 'Millisecond'
      |             name4 = 'ms' ;
      |             fcn4  = '/1000'  ;
      |         case 'Second'
      |             name4 = 's' ;
      |             fcn4  = '' ;
      |         case 'Minute'
      |             name4 = 'min' ;
      |             fcn4  = '*60' ;
      |         case 'Hour'
      |             name4 = 'hr' ;
      |             fcn4  = '*3600' ;
      |     end
      |     expr = [fcn1 fcn2 fcn3 fcn4] ;
      |     %set_param(blk,'func',func) ;
      |     set_param([blk '/conv_fcn'],'expr',expr) ;
      |     str1 = ['% this block of text is updated via dialog callbacks'];
      |     str2 = [char(39) 'horizontalAlignment' char(39) ',' char(39) 'center' char(39) ',' char(39) 'texmode' char(39) ',' char(39) 'on' char(39)] ;
      |     name = [char(39) name1 name2 ' to ' name3 name4 char(39)] ;
      |     str = sprintf('%s\ntext(.5,.5,%s,%s)',str1,name,str2) ;
      |     set_param(blk,'MaskDisplay',str) ;
      | end
      | clear blk value1 value2 value3 value4 expr name1 name2 name3 name4 name fcn1 fcn2 fcn3 fcn4 str1 str2 str
      mask TypeOptions frommfrtime: Millisecond | Second | Minute | Hour
      mask Callback frommfrtime:
      | blk = gcb ;
      | value1 = get_param(blk,'frommfr') ;
      | value2 = get_param(blk,'frommfrtime') ;
      | value3 = get_param(blk,'tomfr') ;
      | value4 = get_param(blk,'tomfrtime') ;
      | if strcmp(get_param(blk,'mfr'),'on')
      |     switch value1
      |         case 'Grams'
      |             name1 = 'g/' ;
      |             fcn1  = 'u(1)*.001' ;
      |         case 'Kilograms'
      |             name1 = 'kg/' ;
      |             fcn1  = 'u(1)' ;
      |         case 'Ounces'
      |             name1 = 'oz/' ;
      |             fcn1  = 'u(1)*.45359237/16' ;
      |         case 'Pounds-Mass'
      |             name1 = 'lbm/' ;
      |             fcn1  = 'u(1)*.45359237' ;
      |         case 'Slugs'
      |             name1 = 'slg/' ;
      |             fcn1  = 'u(1)*14.5939';
      |     end
      |     switch value2
      |         case 'Millisecond'
      |             name2 = 'ms' ;
      |             fcn2  = '*1000'  ;
      |         case 'Second'
      |             name2 = 's' ;
      |             fcn2  = '' ;
      |         case 'Minute'
      |             name2 = 'min' ;
      |             fcn2  = '/60' ;
      |         case 'Hour'
      |             name2 = 'hr' ;
      |             fcn2  = '/3600' ;
      |     end
      |     switch value3
      |         case 'Grams'
      |             name3 = 'g/' ;
      |             fcn3  = '/.001' ;
      |         case 'Kilograms'
      |             name3 = 'kg/' ;
      |             fcn3  = '' ;
      |         case 'Ounces'
      |             name3 = 'oz/' ;
      |             fcn3  = '/.45359237*16' ;
      |         case 'Pounds-Mass'
      |             name3 = 'lbm/' ;
      |             fcn3  = '/.45359237' ;
      |         case 'Slugs'
      |             name3 = 'slg/' ;
      |             fcn3  = '/14.5939';
      |     end
      |     switch value4
      |         case 'Millisecond'
      |             name4 = 'ms' ;
      |             fcn4  = '/1000'  ;
      |         case 'Second'
      |             name4 = 's' ;
      |             fcn4  = '' ;
      |         case 'Minute'
      |             name4 = 'min' ;
      |             fcn4  = '*60' ;
      |         case 'Hour'
      |             name4 = 'hr' ;
      |             fcn4  = '*3600' ;
      |     end
      |     expr = [fcn1 fcn2 fcn3 fcn4] ;
      |     %set_param(blk,'func',func) ;
      |     set_param([blk '/conv_fcn'],'expr',expr) ;
      |     str1 = ['% this block of text is updated via dialog callbacks'];
      |     str2 = [char(39) 'horizontalAlignment' char(39) ',' char(39) 'center' char(39) ',' char(39) 'texmode' char(39) ',' char(39) 'on' char(39)] ;
      |     name = [char(39) name1 name2 ' to ' name3 name4 char(39)] ;
      |     str = sprintf('%s\ntext(.5,.5,%s,%s)',str1,name,str2) ;
      |     set_param(blk,'MaskDisplay',str) ;
      | end
      | clear blk value1 value2 value3 value4 expr name1 name2 name3 name4 name fcn1 fcn2 fcn3 fcn4 str1 str2 str
      mask TypeOptions tomfr: Grams | Kilograms | Ounces | Pounds-Mass | Slugs
      mask Callback tomfr:
      | blk = gcb ;
      | value1 = get_param(blk,'frommfr') ;
      | value2 = get_param(blk,'frommfrtime') ;
      | value3 = get_param(blk,'tomfr') ;
      | value4 = get_param(blk,'tomfrtime') ;
      | if strcmp(get_param(blk,'mfr'),'on')
      |     switch value1
      |         case 'Grams'
      |             name1 = 'g/' ;
      |             fcn1  = 'u(1)*.001' ;
      |         case 'Kilograms'
      |             name1 = 'kg/' ;
      |             fcn1  = 'u(1)' ;
      |         case 'Ounces'
      |             name1 = 'oz/' ;
      |             fcn1  = 'u(1)*.45359237/16' ;
      |         case 'Pounds-Mass'
      |             name1 = 'lbm/' ;
      |             fcn1  = 'u(1)*.45359237' ;
      |         case 'Slugs'
      |             name1 = 'slg/' ;
      |             fcn1  = 'u(1)*14.5939';
      |     end
      |     switch value2
      |         case 'Millisecond'
      |             name2 = 'ms' ;
      |             fcn2  = '*1000'  ;
      |         case 'Second'
      |             name2 = 's' ;
      |             fcn2  = '' ;
      |         case 'Minute'
      |             name2 = 'min' ;
      |             fcn2  = '/60' ;
      |         case 'Hour'
      |             name2 = 'hr' ;
      |             fcn2  = '/3600' ;
      |     end
      |     switch value3
      |         case 'Grams'
      |             name3 = 'g/' ;
      |             fcn3  = '/.001' ;
      |         case 'Kilograms'
      |             name3 = 'kg/' ;
      |             fcn3  = '' ;
      |         case 'Ounces'
      |             name3 = 'oz/' ;
      |             fcn3  = '/.45359237*16' ;
      |         case 'Pounds-Mass'
      |             name3 = 'lbm/' ;
      |             fcn3  = '/.45359237' ;
      |         case 'Slugs'
      |             name3 = 'slg/' ;
      |             fcn3  = '/14.5939';
      |     end
      |     switch value4
      |         case 'Millisecond'
      |             name4 = 'ms' ;
      |             fcn4  = '/1000'  ;
      |         case 'Second'
      |             name4 = 's' ;
      |             fcn4  = '' ;
      |         case 'Minute'
      |             name4 = 'min' ;
      |             fcn4  = '*60' ;
      |         case 'Hour'
      |             name4 = 'hr' ;
      |             fcn4  = '*3600' ;
      |     end
      |     expr = [fcn1 fcn2 fcn3 fcn4] ;
      |     %set_param(blk,'func',func) ;
      |     set_param([blk '/conv_fcn'],'expr',expr) ;
      |     str1 = ['% this block of text is updated via dialog callbacks'];
      |     str2 = [char(39) 'horizontalAlignment' char(39) ',' char(39) 'center' char(39) ',' char(39) 'texmode' char(39) ',' char(39) 'on' char(39)] ;
      |     name = [char(39) name1 name2 ' to ' name3 name4 char(39)] ;
      |     str = sprintf('%s\ntext(.5,.5,%s,%s)',str1,name,str2) ;
      |     set_param(blk,'MaskDisplay',str) ;
      | end
      | clear blk value1 value2 value3 value4 expr name1 name2 name3 name4 name fcn1 fcn2 fcn3 fcn4 str1 str2 str
      mask TypeOptions tomfrtime: Millisecond | Second | Minute | Hour
      mask Callback tomfrtime:
      | blk = gcb ;
      | value1 = get_param(blk,'frommfr') ;
      | value2 = get_param(blk,'frommfrtime') ;
      | value3 = get_param(blk,'tomfr') ;
      | value4 = get_param(blk,'tomfrtime') ;
      | if strcmp(get_param(blk,'mfr'),'on')
      |     switch value1
      |         case 'Grams'
      |             name1 = 'g/' ;
      |             fcn1  = 'u(1)*.001' ;
      |         case 'Kilograms'
      |             name1 = 'kg/' ;
      |             fcn1  = 'u(1)' ;
      |         case 'Ounces'
      |             name1 = 'oz/' ;
      |             fcn1  = 'u(1)*.45359237/16' ;
      |         case 'Pounds-Mass'
      |             name1 = 'lbm/' ;
      |             fcn1  = 'u(1)*.45359237' ;
      |         case 'Slugs'
      |             name1 = 'slg/' ;
      |             fcn1  = 'u(1)*14.5939';
      |     end
      |     switch value2
      |         case 'Millisecond'
      |             name2 = 'ms' ;
      |             fcn2  = '*1000'  ;
      |         case 'Second'
      |             name2 = 's' ;
      |             fcn2  = '' ;
      |         case 'Minute'
      |             name2 = 'min' ;
      |             fcn2  = '/60' ;
      |         case 'Hour'
      |             name2 = 'hr' ;
      |             fcn2  = '/3600' ;
      |     end
      |     switch value3
      |         case 'Grams'
      |             name3 = 'g/' ;
      |             fcn3  = '/.001' ;
      |         case 'Kilograms'
      |             name3 = 'kg/' ;
      |             fcn3  = '' ;
      |         case 'Ounces'
      |             name3 = 'oz/' ;
      |             fcn3  = '/.45359237*16' ;
      |         case 'Pounds-Mass'
      |             name3 = 'lbm/' ;
      |             fcn3  = '/.45359237' ;
      |         case 'Slugs'
      |             name3 = 'slg/' ;
      |             fcn3  = '/14.5939';
      |     end
      |     switch value4
      |         case 'Millisecond'
      |             name4 = 'ms' ;
      |             fcn4  = '/1000'  ;
      |         case 'Second'
      |             name4 = 's' ;
      |             fcn4  = '' ;
      |         case 'Minute'
      |             name4 = 'min' ;
      |             fcn4  = '*60' ;
      |         case 'Hour'
      |             name4 = 'hr' ;
      |             fcn4  = '*3600' ;
      |     end
      |     expr = [fcn1 fcn2 fcn3 fcn4] ;
      |     %set_param(blk,'func',func) ;
      |     set_param([blk '/conv_fcn'],'expr',expr) ;
      |     str1 = ['% this block of text is updated via dialog callbacks'];
      |     str2 = [char(39) 'horizontalAlignment' char(39) ',' char(39) 'center' char(39) ',' char(39) 'texmode' char(39) ',' char(39) 'on' char(39)] ;
      |     name = [char(39) name1 name2 ' to ' name3 name4 char(39)] ;
      |     str = sprintf('%s\ntext(.5,.5,%s,%s)',str1,name,str2) ;
      |     set_param(blk,'MaskDisplay',str) ;
      | end
      | clear blk value1 value2 value3 value4 expr name1 name2 name3 name4 name fcn1 fcn2 fcn3 fcn4 str1 str2 str
      mask Display:
      | % this block of text is updated via dialog callbacks
      | text(.5,.5,'lbm/s to kg/s','horizontalAlignment','center','texmode','on')
  Wf Ramp : simulink/Sources/Ramp  slope=-5  start=0  X0=1.27892
  dTs : Constant  Value=0
  rpm to rad/s : Gain  Gain=2*pi/60
  Engine #1 : Outport
  wires:
  Constant11/1 -> Gain10/1  "FuelLinePres_psi"
  Gain10/1 -> Bus Creator2/1  "FuelLinePres_kPa"
  Gain6/1 -> Unit Conversion 5/1(Signal_in)  "FuelFlow_lb/s"
  Unit Conversion 5/1(Converted Signal Out) -> Manual Switch3/1  "FuelFlow_kgps"
  Electrical/1 -> Bus Selector3/1
  Bus Selector1/2 -> Mux/2  "<Mach>"
  Bus Selector1/1 -> Mux/1  "<altitude_ft>"
  LP CPR/1 -> Bus Creator/2  "BleedAirPres_kPa"
  Isentropic Flow Equation/1 -> Bus Creator/1  "BleedAirTemp_K"
  Bus Selector3/1 -> Subtract/1  "<Left Wing Torq (Nm)>"
  Mission/1 -> Bus Selector1/1
  Manual Switch5/1 -> Bus Creator3/3  "Bleed"
  Bus Creator1/1 -> Bus Creator3/2  "Spools"
  Bus Creator2/1 -> Bus Creator3/1  "Fuel"
  Mission1/1 -> Bus Selector4/1
  Bus Selector4/2 -> Bus Creator4/1, LP CPR/1  "<pres_kPa>"
  Bus Selector4/1 -> Product1/2, Isentropic Flow Equation/1  "<temp_K>"
  dTs/1 -> Mux/3
  Ex Bld/1 -> Mux/7
  LP pwr/1 -> Mux/8
  Demux/1 -> Bus Creator5/1  "Net Thrust (lbf)"
  Demux/2 -> Bus Creator5/2  "Fuel Flow (lbm/s)"
  Demux/3 -> Bus Creator5/3  "LP Speed (rpm)"
  Demux/4 -> Bus Creator5/4  "HP Speed (rpm)"
  Mux/1 -> ?
  Multiport Switch/1 -> Mux/5  "Parm_in"
  [A] -> Multiport Switch/2
  Mode/1 -> Multiport Switch/1, Mux/4  "Mode"
  Demux/5 -> Bus Creator5/5  "Cbld W"
  Demux/6 -> Bus Creator5/6  "Cbld Tt degR"
  Demux/7 -> Bus Creator5/7  "Cbld Pt"
  NL Ramp/1 -> Saturation/1
  Saturation/1 -> [B]
  [B] -> Multiport Switch/3
  Fn Ramp/1 -> Saturation1/1
  Saturation1/1 -> [A]
  Wf Ramp/1 -> Saturation2/1
  Saturation2/1 -> [D]
  RIT Ramp/1 -> Saturation3/1
  Saturation3/1 -> [C]
  Demux/8 -> Bus Creator5/8  "RIT degR"
  Demux/9 -> Bus Creator5/9  "Active Constraint"
  IS Bld/1 -> Mux/6
  [D] -> Multiport Switch/5
  Bus Selector6/1 -> Product/1  "<Left Wing Torq (Nm)>"
  Electrical1/1 -> Bus Selector6/1
  Gain5/1 -> Product/2  "rad/s"
  Product/1 -> "Unit Conversion "/1(Signal_in)
  Manual Switch2/1 -> Mux/9
  HP pwr/1 -> Manual Switch2/1
  "Unit Conversion "/1(Converted Signal Out) -> Manual Switch2/2
  Memory1/1 -> Gain5/1
  Clock/1 -> Defined Fuel Flow Rate/1
  Defined Fuel Flow Rate/1 -> Gain6/1
  Bus Selector4/3 -> Temp inc across fan/1  "<Mach>"
  Temp inc across fan/1 -> Bias/1
  Bias/1 -> Product1/1
  Product1/1 -> Bus Creator4/2  "temp_K"
  Bus Creator4/1 -> Bus Creator3/4  "Bypass"
  Manual Switch4/1 -> rpm to rad/s/1, Gearbox/1(w_engine)  "HPSpoolSpeed_rpm"
  Gearbox/1(w_shaft) -> Scope/1, Bus Creator1/1  "HPSpoolSpeed_rpm"
  Gearbox/2(T_shaft) -> Bus Creator1/2  "HPSpoolTorque_Nm"
  [C] -> Multiport Switch/4
  Bus Creator5/1 -> Bus Selector8/1, Bus Selector7/1, Bus Selector2/1  "Engine1"
  Bus Selector2/1 -> Manual Switch3/2  "<Fuel Flow (lbm/s)>"
  Manual Switch3/1 -> Bus Creator2/2  "FuelFlowNeed_kgps"
  Constant1/1 -> Manual Switch4/2
  Bus Selector7/1 -> Manual Switch4/1  "<HP Speed (rpm)>"
  Bus Selector8/1 -> Unit Conversion 1/1(Signal_in)  "<Cbld Tt degR>"
  Bus Selector8/2 -> Unit Conversion 4/1(Signal_in)  "<Cbld Pt>"
  Unit Conversion 1/1(Converted Signal Out) -> Bus Creator6/1  "BleedAirTemp_K"
  Unit Conversion 4/1(Converted Signal Out) -> Bus Creator6/2  "BleedAirPres_kPa"
  Bus Creator/1 -> Manual Switch5/2  "Bleed"
  Bus Creator6/1 -> Manual Switch5/1
  ? -> Demux/1
  Bus Creator3/1 -> Bus Selector9/1, Engine #1/1
  Bus Selector9/1 -> Memory1/1  "<HPSpoolTorque_Nm>"
  Subtract/1 -> Gearbox/2(T_gen), Engine power/2
  rpm to rad/s/1 -> Engine power/1
  Engine power/1 -> To Workspace/1
  Ground/1 -> Bus Creator3/5  "Oil"
  Constant2/1 -> Subtract/2
